simulink model "OtherControlComponents"  (R2020b)
settings: Solver=FixedStepDiscrete  StartTime=0.0  StopTime=20  FixedStep=1/100  RelTol=1e-3  EnableMultiTasking=on
libraries: pid_lib x4, Electrical_Library x4
settings Model: Creator=ppreethi  LastModifiedBy=YeoJun Choi
settings SolverCC: ExtrapolationOrder=2
settings DataIOCC: LimitDataPoints=on  SaveFormat=Array  SaveOutput=off  SaveTime=off  ReturnWorkspaceOutputs=off
settings OptimizationCC: BlockReduction=off  DefaultParameterBehavior=Inlined  EnhancedBackFolding=on  CachingGlobalReferences=on  LifeSpan=inf  EfficientTunableParamExpr=on
settings DebuggingCC: UnderspecifiedInitializationDetection=Classic  MergeDetectMultiDrivingBlocksExec=none  SolverPrmCheckMsg=warning  BusObjectLabelMismatch=error  StateNameClashWarn=warning  StrictBusMsg=ErrorOnBusTreatedAsVector  NonBusSignalsTreatedAsBus=warning  SFUnexpectedBacktrackingDiag=warning  SFNoUnconditionalDefaultTransitionDiag=warning  SFExecutionAtInitializationDiag=none  ArithmeticOperatorsInVariantConditions=warning
settings HardwareCC: ProdBitPerPointer=32  ProdBitPerSizeT=32  ProdBitPerPtrDiffT=32  ProdLargestAtomicFloat=None  ProdWordSize=32  ProdHWDeviceType=Generic->32-bit x86 compatible
settings ModelReferenceCC: UpdateModelReferenceTargets=IfOutOfDate  ModelReferenceNumInstancesAllowed=Single  PropagateSignalLabelsOutOfModel=off
settings SFSimCC: SimUseLocalCustomCode=off  MATLABDynamicMemAlloc=off  CustomCodeUndefinedFunction=UseInterfaceOnly
settings RTWCC: Description=Embedded Coder  SystemTargetFile=ert.tlc  TLCOptions=-axPCModelStackSizeKB=1024  TemplateMakefile=ert_default_tmf  GenerateReport=on  RTWUseLocalCustomCode=off  IncludeHyperlinkInReport=on  LaunchReport=on  RTWCompilerOptimization=on
settings CodeAppCC: IgnoreCustomStorageClasses=off  StateflowObjectComments=on
settings ERTTargetCC: MultiwordLength=2048  GenerateSampleERTMain=on  IncludeMdlTerminateFcn=off  SuppressErrorStatus=on  SupportAbsoluteTime=off  SupportNonFinite=off  SupportComplex=off  InlinedParameterPlacement=NonHierarchical  ERTCustomFileTemplate=example_file_process.tlc  ConvertIfToSwitch=off  SuppressUnreachableDefaultCases=off
settings ConfigComp: CovMetricSettings=dw  CovSaveCumulativeToWorkspaceVar=on  CovSaveSingleToWorkspaceVar=on  CovExternalEMLEnable=off  CovSFcnEnable=off  DVModelCoverageObjectives=MCDC  DVMaxTestCaseSteps=500  DVTestSuiteOptimization=CombinedObjectives (Nonlinear Extended)  DVIncludeRelationalBoundary=on  DVDetectOutOfBounds=on  DVDesignMinMaxCheck=on  DVSaveHarnessModel=on  DVModelReferenceHarness=on
settings SimscapeCC: SimscapeNormalizeSystem=off
settings ConfigurationSet: Description=SimMechanics 2G
settings ExplorerConfigSet: InternalSimMechanicsExplorerSettings="<ExplorerConfiguration><canonicalview>default</canonicalview><AnimationSetting><BasePlaybackSpeed>1.0</BasePlaybackSpeed><PlaybackSpeedFactor>1.0</PlaybackSpeedFactor></AnimationSetting><TilePanel><TileInfo><Tiles Columns=\"1\" Count=\"1\" Rows=\"1\"><Column Left=\"2\" Weight=\"1\"/><Column Left=\"1669\"/><Row Top=\"2\" Weight=\"1\"/><Row Top=\"1032\"/><Tile Height=\"1\" Width=\"1\" X=\"0\" Y=\"0\"/></Tiles></TileInfo><SceneInfo><SceneViewer><BGColor><R>1</R><G>1</G><B>1</B></BGColor><Camera><Position><X>-0.98734234069472837</X><Y>-2.5766196877608176</Y><Z>-0.21434917441758128</Z></Position><Center><X>-0.36548137966941641</X><Y>0.086653013342029503</Y><Z>0.52407155472837563</Z></Center><Up><X>-0.18648657026384141</X><Y>0.30268994651916503</Y><Z>-0.93466654769893953</Z></Up><Left>-0.88113891027964153</Left><Right>0.88113891027964153</Right><Bottom>-0.94141860281001366</Bottom><Top>0.94141860281001366</Top></Camera></SceneViewer></SceneInfo></TilePanel></ExplorerConfiguration>"

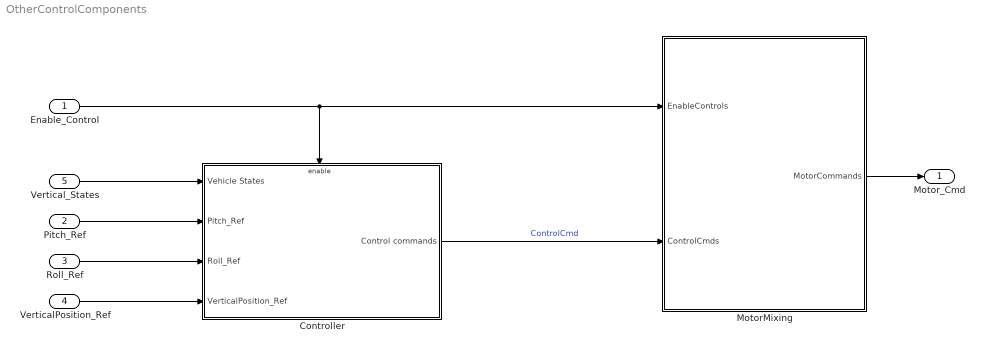
== system OtherControlComponents ==
  Enable_Control : Inport  OutDataTypeStr=boolean  PortDimensions=1  SampleTime=[0.01,0]
  Pitch_Ref : Inport  Port=2  OutDataTypeStr=single  PortDimensions=1  SampleTime=[0.01,0]
  Roll_Ref : Inport  Port=3  OutDataTypeStr=single  PortDimensions=1  SampleTime=[0.01,0]
  VerticalPosition_Ref : Inport  Port=4  OutDataTypeStr=single  PortDimensions=1  SampleTime=[0.01,0]
  Vertical_States : Inport  Port=5  OutDataTypeStr=Bus: NavigationStates  PortDimensions=1  SampleTime=[0.01,0]  BusOutputAsStruct=on
  Controller : Subsystem
  MotorMixing : Subsystem
  Motor_Cmd : Outport  OutDataTypeStr=Bus: MotorCommands
  wires:
  Vertical_States/1 -> Controller/1(Vehicle States)
  Enable_Control/1 -> MotorMixing/1(EnableControls), Controller/Enable
  VerticalPosition_Ref/1 -> Controller/4(VerticalPosition_Ref)
  Roll_Ref/1 -> Controller/3(Roll_Ref)
  Pitch_Ref/1 -> Controller/2(Pitch_Ref)
  MotorMixing/1(MotorCommands) -> Motor_Cmd/1
  Controller/1(Control commands) -> MotorMixing/2(ControlCmds)  "ControlCmd"

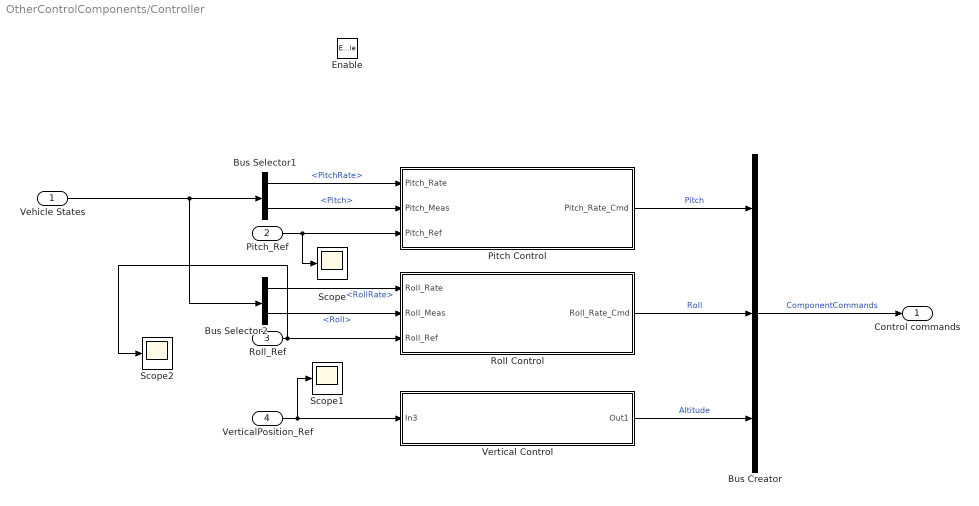
== system OtherControlComponents/Controller ==
  Vehicle States : Inport  OutDataTypeStr=Bus: NavigationStates
  Pitch_Ref : Inport  Port=2
  Roll_Ref : Inport  Port=3
  VerticalPosition_Ref : Inport  Port=4
  Enable : EnablePort
  Bus Creator : BusCreator  Inputs=3  OutDataTypeStr=Bus: ControllerBus  NonVirtualBus=on
  Bus Selector1 : BusSelector  OutputSignals=PitchRate,Pitch
  Bus Selector2 : BusSelector  OutputSignals=RollRate,Roll
  Pitch Control : Subsystem
  Roll Control : Subsystem
  Scope : Scope
  Scope1 : Scope
  Scope2 : Scope
  Vertical Control : Subsystem
  Control commands : Outport
  wires:
  Bus Selector2/1 -> Roll Control/1(Roll_Rate)  "<RollRate>"
  Bus Selector2/2 -> Roll Control/2(Roll_Meas)  "<Roll>"
  Bus Selector1/1 -> Pitch Control/1(Pitch_Rate)  "<PitchRate>"
  Bus Selector1/2 -> Pitch Control/2(Pitch_Meas)  "<Pitch>"
  VerticalPosition_Ref/1 -> Scope1/1, Vertical Control/1(In3)
  Roll_Ref/1 -> Scope2/1, Roll Control/3(Roll_Ref)
  Pitch_Ref/1 -> Scope/1, Pitch Control/3(Pitch_Ref)
  Bus Creator/1 -> Control commands/1  "ComponentCommands"
  Pitch Control/1(Pitch_Rate_Cmd) -> Bus Creator/1  "Pitch"
  Roll Control/1(Roll_Rate_Cmd) -> Bus Creator/2  "Roll"
  Vertical Control/1(Out1) -> Bus Creator/3  "Altitude"
  Vehicle States/1 -> Bus Selector1/1, Bus Selector2/1

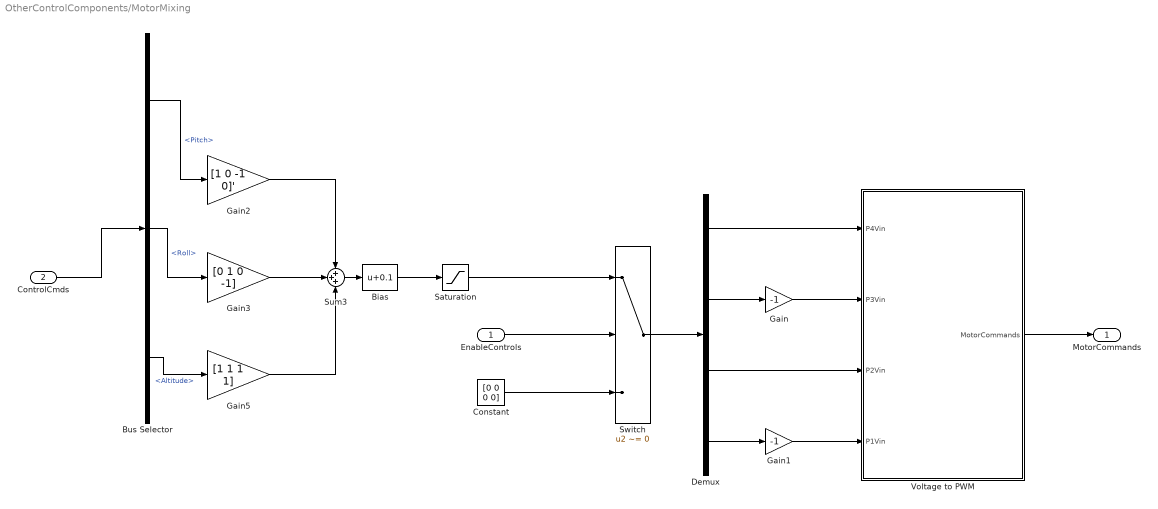
== system OtherControlComponents/MotorMixing ==
  EnableControls : Inport
  ControlCmds : Inport  Port=2  OutDataTypeStr=Bus: ControllerBus
  Bias : Bias  Bias=0.1
  Bus Selector : BusSelector  OutputSignals=Pitch,Roll,Altitude
  Constant : Constant  Value=[0 0 0 0]  OutDataTypeStr=single
  Demux : Demux
  Gain : Gain  Gain=-1
  Gain1 : Gain  Gain=-1
  Gain2 : Gain  Gain=[1 0 -1 0]'
  Gain3 : Gain  Gain=[0 1 0 -1]
  Gain5 : Gain  Gain=[1 1 1 1]
  Saturation : Saturate  UpperLimit=4  LowerLimit=-4
  Sum3 : Sum  Inputs=+++
  Switch : Switch  Criteria=u2 ~= 0
  Voltage to PWM : Subsystem
  MotorCommands : Outport
  wires:
  Bus Selector/3 -> Gain5/1  "<Altitude>"
  Bus Selector/1 -> Gain2/1  "<Pitch>"
  Bus Selector/2 -> Gain3/1  "<Roll>"
  Demux/2 -> Gain/1
  Demux/4 -> Gain1/1
  Demux/1 -> Voltage to PWM/1(P4Vin)
  Demux/3 -> Voltage to PWM/3(P2Vin)
  Gain/1 -> Voltage to PWM/2(P3Vin)
  Gain1/1 -> Voltage to PWM/4(P1Vin)
  Voltage to PWM/1(MotorCommands) -> MotorCommands/1
  ControlCmds/1 -> Bus Selector/1
  Bias/1 -> Saturation/1
  Saturation/1 -> Switch/1
  Sum3/1 -> Bias/1
  Gain5/1 -> Sum3/3
  Gain2/1 -> Sum3/1
  Gain3/1 -> Sum3/2
  Switch/1 -> Demux/1
  Constant/1 -> Switch/3
  EnableControls/1 -> Switch/2

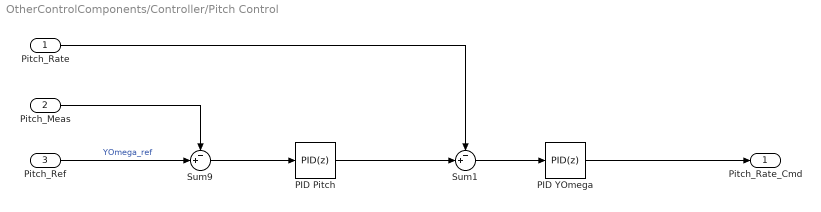
== system OtherControlComponents/Controller/Pitch Control ==
  Pitch_Rate : Inport
  Pitch_Meas : Inport  Port=2
  Pitch_Ref : Inport  Port=3
  " PID Pitch" : pid_lib/PID Controller  Controller=PID  Form=Parallel  TimeDomain=Discrete-time  UseExternalTs=off  SampleTime=0.01  IntegratorMethod=Forward Euler  FilterMethod=Forward Euler  ControllerParametersSource=internal  P=0.161968253586349  I=0.0142135445800466  D=-0.00457687845999478  UseFilter=on  N=11.2352356409556  TunerSelectOption=Transfer Function Based (PID Tuner App)  InitialConditionSource=internal  InitialConditionForIntegrator=0  InitialConditionForFilter=0  DifferentiatorICPrevScaledInput=0  ExternalReset=none  TrackingMode=off  Kt=1  LimitOutput=off  SatLimitsSource=internal  UpperSaturationLimit=inf  LowerSaturationLimit=-inf  LinearizeAsGain=on  AntiWindupMode=none  Kb=1  POutMin=[]  POutMax=[]  IOutMin=[]  IOutMax=[]  DOutMin=[]  DOutMax=[]  NOutMin=[]  NOutMax=[]  SumOutMin=[]  SumOutMax=[]  SaturationOutMin=[]  SaturationOutMax=[]  PParamMin=[]  PParamMax=[]  IParamMin=[]  IParamMax=[]  DParamMin=[]  DParamMax=[]  NParamMin=[]  NParamMax=[]  KbParamMin=[]  KbParamMax=[]  KtParamMin=[]  KtParamMax=[]  KbOutMin=[]  KbOutMax=[]  KtOutMin=[]  KtOutMax=[]  IntegratorOutMin=[]  IntegratorOutMax=[]  FilterOutMin=[]  FilterOutMax=[]  SumI1OutMin=[]  SumI1OutMax=[]  SumI2OutMin=[]  SumI2OutMax=[]  SumI3OutMin=[]  SumI3OutMax=[]  SumI4OutMin=[]  SumI4OutMax=[]  SumDOutMin=[]  SumDOutMax=[]  DifferentiatorOutMin=[]  DifferentiatorOutMax=[]  FilterDiffOutCoefMin=[]  FilterDiffOutCoefMax=[]  ReciprocalOutMin=[]  ReciprocalOutMax=[]  SumDenOutMin=[]  SumDenOutMax=[]  SumNumOutMin=[]  SumNumOutMax=[]  DivideOutMin=[]  DivideOutMax=[]  UdiffTsProdOutMin=[]  UdiffTsProdOutMax=[]  NTsProdOutMin=[]  NTsProdOutMax=[]  UintegralTsProdOutMin=[]  UintegralTsProdOutMax=[]  UngainTsProdOutMin=[]  UngainTsProdOutMax=[]  IntegratorContinuousStateAttributes=''  IntegratorStateMustResolveToSignalObject=off  IntegratorRTWStateStorageClass=Auto  FilterContinuousStateAttributes=''  FilterStateMustResolveToSignalObject=off  FilterRTWStateStorageClass=Auto  ParallelPVariant=InternalParameters  IdealPVariant=Disabled  IVariant=InternalParameters  DVariant=InternalParameters  IntegratorVariant=Discrete  SatVariant=Disabled  AWVariant=Passthrough  PCopyVariant=Disabled  TRVariant=Disabled  FdbkBlocksVariant=Forward  IdealPFdbkVariant=Disabled  SatFdbkVariant=Disabled  DerivativeFilterVariant=ForwardEulerFilter  NVariant=InternalParameters  NCopyVariant=Disabled  FilterICVariant=InternalICsFilter  IntegratorICVariant=InternalICs  ExternalResetVariant=Disabled  TRSumVariant=Passthrough  SumFdbkVariant=Disabled  SumVariant=Sum_PID  TsampFilterVariant=InternalTs  TsampNgainVariant=Passthrough  TsampIntegralVariant=Passthrough  ExternalSaturationOutDataTypeStr=Inherit: Same as second input
  PID YOmega : pid_lib/PID Controller  Controller=PID  Form=Parallel  TimeDomain=Discrete-time  UseExternalTs=off  SampleTime=0.01  IntegratorMethod=Forward Euler  FilterMethod=Forward Euler  ControllerParametersSource=internal  P=-0.617679800762959  I=-0.121328919441601  D=-0.0496012913890723  UseFilter=on  N=76.7547894350947  TunerSelectOption=Transfer Function Based (PID Tuner App)  InitialConditionSource=internal  InitialConditionForIntegrator=0  InitialConditionForFilter=0  DifferentiatorICPrevScaledInput=0  ExternalReset=none  TrackingMode=off  Kt=1  LimitOutput=off  SatLimitsSource=internal  UpperSaturationLimit=inf  LowerSaturationLimit=-inf  LinearizeAsGain=on  AntiWindupMode=none  Kb=1  POutMin=[]  POutMax=[]  IOutMin=[]  IOutMax=[]  DOutMin=[]  DOutMax=[]  NOutMin=[]  NOutMax=[]  SumOutMin=[]  SumOutMax=[]  SaturationOutMin=[]  SaturationOutMax=[]  PParamMin=[]  PParamMax=[]  IParamMin=[]  IParamMax=[]  DParamMin=[]  DParamMax=[]  NParamMin=[]  NParamMax=[]  KbParamMin=[]  KbParamMax=[]  KtParamMin=[]  KtParamMax=[]  KbOutMin=[]  KbOutMax=[]  KtOutMin=[]  KtOutMax=[]  IntegratorOutMin=[]  IntegratorOutMax=[]  FilterOutMin=[]  FilterOutMax=[]  SumI1OutMin=[]  SumI1OutMax=[]  SumI2OutMin=[]  SumI2OutMax=[]  SumI3OutMin=[]  SumI3OutMax=[]  SumI4OutMin=[]  SumI4OutMax=[]  SumDOutMin=[]  SumDOutMax=[]  DifferentiatorOutMin=[]  DifferentiatorOutMax=[]  FilterDiffOutCoefMin=[]  FilterDiffOutCoefMax=[]  ReciprocalOutMin=[]  ReciprocalOutMax=[]  SumDenOutMin=[]  SumDenOutMax=[]  SumNumOutMin=[]  SumNumOutMax=[]  DivideOutMin=[]  DivideOutMax=[]  UdiffTsProdOutMin=[]  UdiffTsProdOutMax=[]  NTsProdOutMin=[]  NTsProdOutMax=[]  UintegralTsProdOutMin=[]  UintegralTsProdOutMax=[]  UngainTsProdOutMin=[]  UngainTsProdOutMax=[]  IntegratorContinuousStateAttributes=''  IntegratorStateMustResolveToSignalObject=off  IntegratorRTWStateStorageClass=Auto  FilterContinuousStateAttributes=''  FilterStateMustResolveToSignalObject=off  FilterRTWStateStorageClass=Auto  ParallelPVariant=InternalParameters  IdealPVariant=Disabled  IVariant=InternalParameters  DVariant=InternalParameters  IntegratorVariant=Discrete  SatVariant=Disabled  AWVariant=Passthrough  PCopyVariant=Disabled  TRVariant=Disabled  FdbkBlocksVariant=Forward  IdealPFdbkVariant=Disabled  SatFdbkVariant=Disabled  DerivativeFilterVariant=ForwardEulerFilter  NVariant=InternalParameters  NCopyVariant=Disabled  FilterICVariant=InternalICsFilter  IntegratorICVariant=InternalICs  ExternalResetVariant=Disabled  TRSumVariant=Passthrough  SumFdbkVariant=Disabled  SumVariant=Sum_PID  TsampFilterVariant=InternalTs  TsampNgainVariant=Passthrough  TsampIntegralVariant=Passthrough  ExternalSaturationOutDataTypeStr=Inherit: Same as second input
  Sum1 : Sum  Inputs=-+|
  Sum9 : Sum  Inputs=-+|
  Pitch_Rate_Cmd : Outport
  wires:
  Sum1/1 -> PID YOmega/1
  Pitch_Rate/1 -> Sum1/1
  Pitch_Ref/1 -> Sum9/2  "YOmega_ref"
  Sum9/1 -> " PID Pitch"/1
  PID YOmega/1 -> Pitch_Rate_Cmd/1
  " PID Pitch"/1 -> Sum1/2
  Pitch_Meas/1 -> Sum9/1

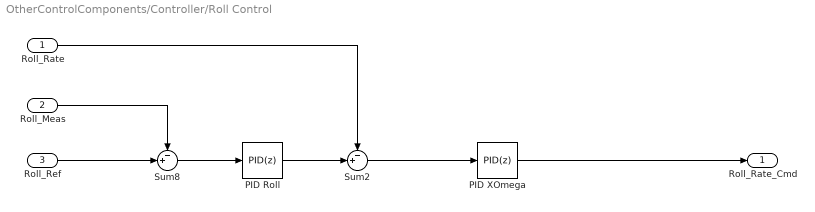
== system OtherControlComponents/Controller/Roll Control ==
  Roll_Rate : Inport
  Roll_Meas : Inport  Port=2
  Roll_Ref : Inport  Port=3
  " PID Roll" : pid_lib/PID Controller  Controller=PID  Form=Parallel  TimeDomain=Discrete-time  UseExternalTs=off  SampleTime=0.01  IntegratorMethod=Forward Euler  FilterMethod=Forward Euler  ControllerParametersSource=internal  P=0.163786869100367  I=0.0131100645340934  D=-0.00552577256315964  UseFilter=on  N=8.72815063273421  TunerSelectOption=Transfer Function Based (PID Tuner App)  InitialConditionSource=internal  InitialConditionForIntegrator=0  InitialConditionForFilter=0  DifferentiatorICPrevScaledInput=0  ExternalReset=none  TrackingMode=off  Kt=1  LimitOutput=off  SatLimitsSource=internal  UpperSaturationLimit=inf  LowerSaturationLimit=-inf  LinearizeAsGain=on  AntiWindupMode=none  Kb=1  POutMin=[]  POutMax=[]  IOutMin=[]  IOutMax=[]  DOutMin=[]  DOutMax=[]  NOutMin=[]  NOutMax=[]  SumOutMin=[]  SumOutMax=[]  SaturationOutMin=[]  SaturationOutMax=[]  PParamMin=[]  PParamMax=[]  IParamMin=[]  IParamMax=[]  DParamMin=[]  DParamMax=[]  NParamMin=[]  NParamMax=[]  KbParamMin=[]  KbParamMax=[]  KtParamMin=[]  KtParamMax=[]  KbOutMin=[]  KbOutMax=[]  KtOutMin=[]  KtOutMax=[]  IntegratorOutMin=[]  IntegratorOutMax=[]  FilterOutMin=[]  FilterOutMax=[]  SumI1OutMin=[]  SumI1OutMax=[]  SumI2OutMin=[]  SumI2OutMax=[]  SumI3OutMin=[]  SumI3OutMax=[]  SumI4OutMin=[]  SumI4OutMax=[]  SumDOutMin=[]  SumDOutMax=[]  DifferentiatorOutMin=[]  DifferentiatorOutMax=[]  FilterDiffOutCoefMin=[]  FilterDiffOutCoefMax=[]  ReciprocalOutMin=[]  ReciprocalOutMax=[]  SumDenOutMin=[]  SumDenOutMax=[]  SumNumOutMin=[]  SumNumOutMax=[]  DivideOutMin=[]  DivideOutMax=[]  UdiffTsProdOutMin=[]  UdiffTsProdOutMax=[]  NTsProdOutMin=[]  NTsProdOutMax=[]  UintegralTsProdOutMin=[]  UintegralTsProdOutMax=[]  UngainTsProdOutMin=[]  UngainTsProdOutMax=[]  IntegratorContinuousStateAttributes=''  IntegratorStateMustResolveToSignalObject=off  IntegratorRTWStateStorageClass=Auto  FilterContinuousStateAttributes=''  FilterStateMustResolveToSignalObject=off  FilterRTWStateStorageClass=Auto  ParallelPVariant=InternalParameters  IdealPVariant=Disabled  IVariant=InternalParameters  DVariant=InternalParameters  IntegratorVariant=Discrete  SatVariant=Disabled  AWVariant=Passthrough  PCopyVariant=Disabled  TRVariant=Disabled  FdbkBlocksVariant=Forward  IdealPFdbkVariant=Disabled  SatFdbkVariant=Disabled  DerivativeFilterVariant=ForwardEulerFilter  NVariant=InternalParameters  NCopyVariant=Disabled  FilterICVariant=InternalICsFilter  IntegratorICVariant=InternalICs  ExternalResetVariant=Disabled  TRSumVariant=Passthrough  SumFdbkVariant=Disabled  SumVariant=Sum_PID  TsampFilterVariant=InternalTs  TsampNgainVariant=Passthrough  TsampIntegralVariant=Passthrough  ExternalSaturationOutDataTypeStr=Inherit: Same as second input
  " PID XOmega" : pid_lib/PID Controller  Controller=PID  Form=Parallel  TimeDomain=Discrete-time  UseExternalTs=off  SampleTime=0.01  IntegratorMethod=Forward Euler  FilterMethod=Forward Euler  ControllerParametersSource=internal  P=-0.464796681482622  I=-0.0944724960148982  D=-0.0568842678742738  UseFilter=on  N=78.8436382942649  TunerSelectOption=Transfer Function Based (PID Tuner App)  InitialConditionSource=internal  InitialConditionForIntegrator=0  InitialConditionForFilter=0  DifferentiatorICPrevScaledInput=0  ExternalReset=none  TrackingMode=off  Kt=1  LimitOutput=off  SatLimitsSource=internal  UpperSaturationLimit=inf  LowerSaturationLimit=-inf  LinearizeAsGain=on  AntiWindupMode=none  Kb=1  POutMin=[]  POutMax=[]  IOutMin=[]  IOutMax=[]  DOutMin=[]  DOutMax=[]  NOutMin=[]  NOutMax=[]  SumOutMin=[]  SumOutMax=[]  SaturationOutMin=[]  SaturationOutMax=[]  PParamMin=[]  PParamMax=[]  IParamMin=[]  IParamMax=[]  DParamMin=[]  DParamMax=[]  NParamMin=[]  NParamMax=[]  KbParamMin=[]  KbParamMax=[]  KtParamMin=[]  KtParamMax=[]  KbOutMin=[]  KbOutMax=[]  KtOutMin=[]  KtOutMax=[]  IntegratorOutMin=[]  IntegratorOutMax=[]  FilterOutMin=[]  FilterOutMax=[]  SumI1OutMin=[]  SumI1OutMax=[]  SumI2OutMin=[]  SumI2OutMax=[]  SumI3OutMin=[]  SumI3OutMax=[]  SumI4OutMin=[]  SumI4OutMax=[]  SumDOutMin=[]  SumDOutMax=[]  DifferentiatorOutMin=[]  DifferentiatorOutMax=[]  FilterDiffOutCoefMin=[]  FilterDiffOutCoefMax=[]  ReciprocalOutMin=[]  ReciprocalOutMax=[]  SumDenOutMin=[]  SumDenOutMax=[]  SumNumOutMin=[]  SumNumOutMax=[]  DivideOutMin=[]  DivideOutMax=[]  UdiffTsProdOutMin=[]  UdiffTsProdOutMax=[]  NTsProdOutMin=[]  NTsProdOutMax=[]  UintegralTsProdOutMin=[]  UintegralTsProdOutMax=[]  UngainTsProdOutMin=[]  UngainTsProdOutMax=[]  IntegratorContinuousStateAttributes=''  IntegratorStateMustResolveToSignalObject=off  IntegratorRTWStateStorageClass=Auto  FilterContinuousStateAttributes=''  FilterStateMustResolveToSignalObject=off  FilterRTWStateStorageClass=Auto  ParallelPVariant=InternalParameters  IdealPVariant=Disabled  IVariant=InternalParameters  DVariant=InternalParameters  IntegratorVariant=Discrete  SatVariant=Disabled  AWVariant=Passthrough  PCopyVariant=Disabled  TRVariant=Disabled  FdbkBlocksVariant=Forward  IdealPFdbkVariant=Disabled  SatFdbkVariant=Disabled  DerivativeFilterVariant=ForwardEulerFilter  NVariant=InternalParameters  NCopyVariant=Disabled  FilterICVariant=InternalICsFilter  IntegratorICVariant=InternalICs  ExternalResetVariant=Disabled  TRSumVariant=Passthrough  SumFdbkVariant=Disabled  SumVariant=Sum_PID  TsampFilterVariant=InternalTs  TsampNgainVariant=Passthrough  TsampIntegralVariant=Passthrough  ExternalSaturationOutDataTypeStr=Inherit: Same as second input
  Sum2 : Sum  Inputs=-+|
  Sum8 : Sum  Inputs=-+|
  Roll_Rate_Cmd : Outport
  wires:
  Roll_Rate/1 -> Sum2/1
  Roll_Meas/1 -> Sum8/1
  Roll_Ref/1 -> Sum8/2
  Sum2/1 -> " PID XOmega"/1
  " PID Roll"/1 -> Sum2/2
  Sum8/1 -> " PID Roll"/1
  " PID XOmega"/1 -> Roll_Rate_Cmd/1

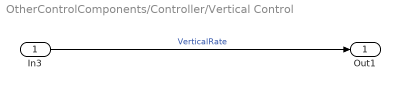
== system OtherControlComponents/Controller/Vertical Control ==
  In3 : Inport
  Out1 : Outport
  wires:
  In3/1 -> Out1/1  "VerticalRate"

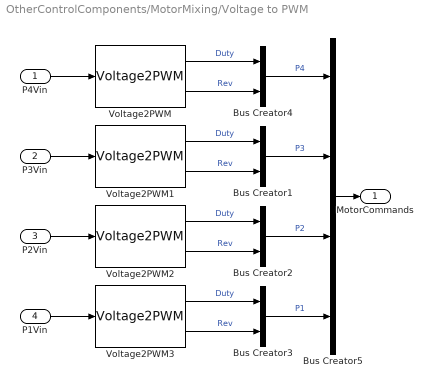
== system OtherControlComponents/MotorMixing/Voltage to PWM ==
  P4Vin : Inport
  P3Vin : Inport  Port=2
  P2Vin : Inport  Port=3
  P1Vin : Inport  Port=4
  Bus Creator{1..4} (4 alike) : BusCreator  Inputs=2  OutDataTypeStr=Bus: PWMBus
  Bus Creator5 : BusCreator  Inputs=4  OutDataTypeStr=Bus: MotorCommands
  Voltage2PWM{,1..3} (4 alike) : Electrical_Library/Voltage2PWM  SystemSampleTime=-1  VariantActivationTime=update diagram  Latency=0  AutoFrameSizeCalculation=off
  MotorCommands : Outport  OutDataTypeStr=Bus: MotorCommands
  wires:
  P4Vin/1 -> Voltage2PWM/1
  P2Vin/1 -> Voltage2PWM2/1
  P1Vin/1 -> Voltage2PWM3/1
  P3Vin/1 -> Voltage2PWM1/1
  Bus Creator4/1 -> Bus Creator5/1  "P4"
  Voltage2PWM/1 -> Bus Creator4/1  "Duty"
  Voltage2PWM/2 -> Bus Creator4/2  "Rev"
  Bus Creator2/1 -> Bus Creator5/3  "P2"
  Bus Creator3/1 -> Bus Creator5/4  "P1"
  Bus Creator1/1 -> Bus Creator5/2  "P3"
  Voltage2PWM1/1 -> Bus Creator1/1  "Duty"
  Voltage2PWM1/2 -> Bus Creator1/2  "Rev"
  Voltage2PWM2/1 -> Bus Creator2/1  "Duty"
  Voltage2PWM2/2 -> Bus Creator2/2  "Rev"
  Voltage2PWM3/1 -> Bus Creator3/1  "Duty"
  Voltage2PWM3/2 -> Bus Creator3/2  "Rev"
  Bus Creator5/1 -> MotorCommands/1
